simulink model "BangBangHysteresisModel"  (R2024a)
settings: Solver=FixedStepAuto  StartTime=0.0  StopTime=tFinal_s  FixedStep=deltaT_s  RelTol=1e-3  EnableMultiTasking=on
values from neighbouring files (symbols this model uses):
  deadbandSize_C = 0.01    [Step04_BangBangHysteresisSetupModel.m]
  u_ON = 1    [Step04_BangBangHysteresisSetupModel.m]
libraries: TemperatureControlLibrary x2
settings Model: SimulationMode=external  ExtModeTrigDuration=2  Creator=Christopher  LastModifiedBy=chris
settings SolverCC: AlgebraicLoopSolver=TrustRegion  AutoInsertRateTranBlk=on
settings DataIOCC: LimitDataPoints=on  StreamToWorkspace=on  ReturnWorkspaceOutputs=off
settings OptimizationCC: LifeSpan=1  MaxStackSize=64
settings DebuggingCC: UnconnectedInputMsg=warning  UnconnectedOutputMsg=warning  UnconnectedLineMsg=warning  AllowSymbolicDim=off  SFUnexpectedBacktrackingDiag=warning  SFNoUnconditionalDefaultTransitionDiag=warning  SFExecutionAtInitializationDiag=none  ArithmeticOperatorsInVariantConditions=warning
settings HardwareCC: ProdBitPerInt=16  ProdBitPerPointer=16  ProdBitPerSizeT=16  ProdBitPerPtrDiffT=16  ProdLargestAtomicFloat=None  ProdWordSize=8  ProdHWDeviceType=Atmel->AVR
settings ModelReferenceCC: EnableRefExpFcnMdlSchedulingChecks=on  PropagateSignalLabelsOutOfModel=off
settings SFSimCC: SimUseLocalCustomCode=off  CustomCodeUndefinedFunction=UseInterfaceOnly
settings RTWCC: Description=Embedded Coder  SystemTargetFile=ert.tlc  HardwareBoard=Arduino Nano 3.0  TemplateMakefile=ert_default_tmf  RTWVerbose=off  RTWUseLocalCustomCode=off  Toolchain=Arduino AVR  BuildConfiguration=Faster Runs  GPUComputeCapability=3.5
settings CodeAppCC: MangleLength=10  StateflowObjectComments=on
settings ERTTargetCC: MultiwordLength=2048  ERTCustomFileBanners=off  SupportContinuousTime=on  SupportNonInlinedSFcns=on  RemoveResetFunc=off  SupportVariableSizeSignals=on  ModelStepFunctionPrototypeControlCompliant=off  ExtMode=on  ExtModeTransport=3  ExtModeStaticAlloc=on  ExtModeAutomaticAllocSize=off  ExtModeStaticAllocSize=250  ExtModeMexFile=ext_xcp  ExtModeMexArgs='127.0.0.1' 0 17725  ExtModeIntrfLevel=Level2 - Open  ERTSrcFileBannerTemplate=codertarget_code_template.cgt  ERTHdrFileBannerTemplate=codertarget_code_template.cgt  ERTDataSrcFileTemplate=codertarget_code_template.cgt  ERTDataHdrFileTemplate=codertarget_code_template.cgt  ConvertIfToSwitch=off  SuppressUnreachableDefaultCases=off
settings ConfigComp: CovMetricSettings=dw  CovSaveCumulativeToWorkspaceVar=on  CovSaveSingleToWorkspaceVar=on  CovExternalEMLEnable=off

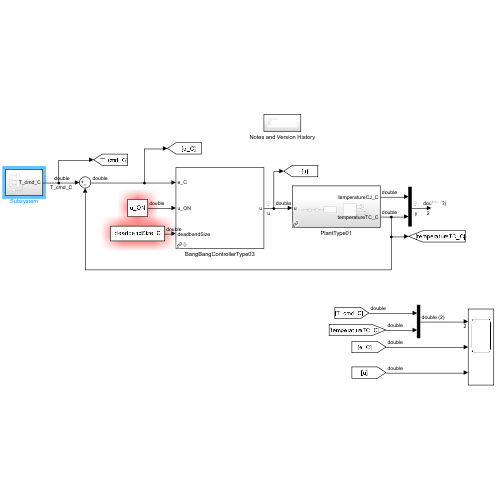
[thumbnail: Simulink's stored preview of the top-level diagram]
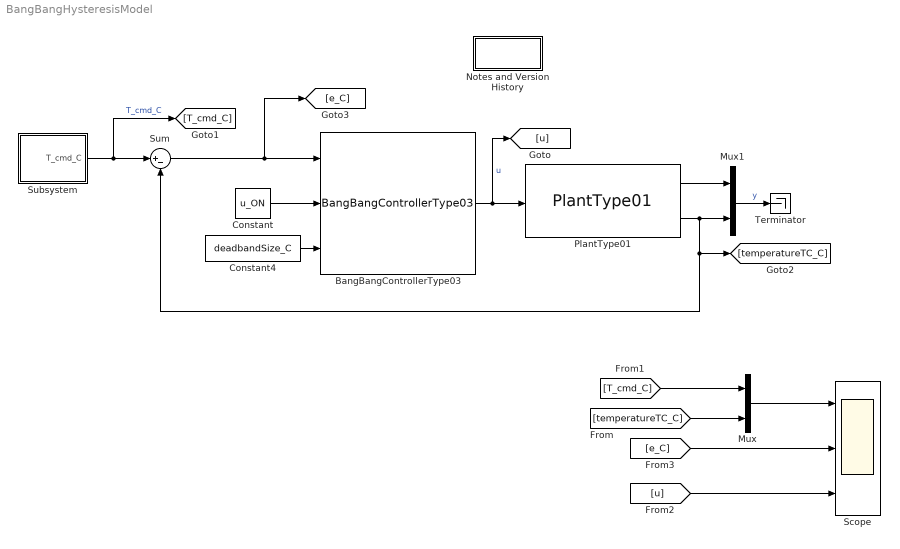
== system BangBangHysteresisModel ==
  BangBangControllerType03 : TemperatureControlLibrary/BangBangControllerType03
  Constant : Constant  Value=u_ON
  Constant4 : Constant  Value=deadbandSize_C
  Mux : Mux  Inputs=2
  Mux1 : Mux  Inputs=2
  Notes and Version History : Subsystem
  PlantType01 : TemperatureControlLibrary/PlantType01  SystemSampleTime=-1  VariantActivationTime=update diagram  AllowFlexibleInterface=on  Latency=0  AutoFrameSizeCalculation=off
  Scope : Scope  NumInputPorts=3
  Subsystem : Subsystem
  Sum : Sum  Inputs=|+-
  Terminator : Terminator
  wires:
  Mux1/1 -> Terminator/1  "y"
  [u] -> Scope/3
  PlantType01/1 -> Mux1/1
  PlantType01/2 -> Sum/2, [temperatureTC_C], Mux1/2
  [T_cmd_C] -> Mux/1
  [temperatureTC_C] -> Mux/2
  Mux/1 -> Scope/1
  Subsystem/1(T_cmd_C) -> Sum/1, [T_cmd_C]  "T_cmd_C"
  Sum/1 -> [e_C], BangBangControllerType03/1
  Constant/1 -> BangBangControllerType03/2
  Constant4/1 -> BangBangControllerType03/3
  [e_C] -> Scope/2
  BangBangControllerType03/1 -> [u], PlantType01/1  "u"

== system BangBangHysteresisModel/Notes and Version History ==
  note: Bang/bang temperature control.
      |
      | Measure temperature using a MAX31856 via SPI.
      |
      | Actuator is a heater.
      |
      | Christopher Lum
      | lum@uw.edu
      |
      | Version History
      | 02/01/25: Created

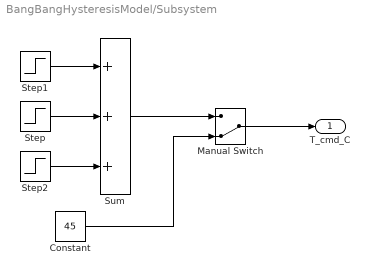
== system BangBangHysteresisModel/Subsystem ==
  Constant : Constant  Value=45
  Manual Switch : ManualSwitch  CurrentSetting=0
  Step : Step  Time=2.5*60  After=-5  SampleTime=0
  Step1 : Step  Time=5  After=45  SampleTime=0
  Step2 : Step  Time=250  After=10  SampleTime=0
  Sum : Sum  Inputs=+++
  T_cmd_C : Outport
  wires:
  Step1/1 -> Sum/1
  Step/1 -> Sum/2
  Sum/1 -> Manual Switch/1
  Step2/1 -> Sum/3
  Constant/1 -> Manual Switch/2
  Manual Switch/1 -> T_cmd_C/1
